simulink model "ppi_ctrl"  (R2020b)
settings: Solver=VariableStepAuto  StartTime=0.0  StopTime=10.0  RelTol=1e-3
values from neighbouring files (symbols this model uses):
  Ka = M_    [ppi_tuning.m]
  Kd = deltad1(2)*M_    [ppi_tuning.m]
  Ki = deltad1(3)*M_    [ppi_tuning.m]
  Kp = deltad2(1)/deltad1(3)    [ppi_tuning.m]    (also in script_ppi.m = double(Kp))
  q0 = [0 0 0 0]'    [script_ppi.m]
  traj_switch = 0    [script_ppi.m]
settings Model: Creator=lucas  LastModifiedBy=lucas

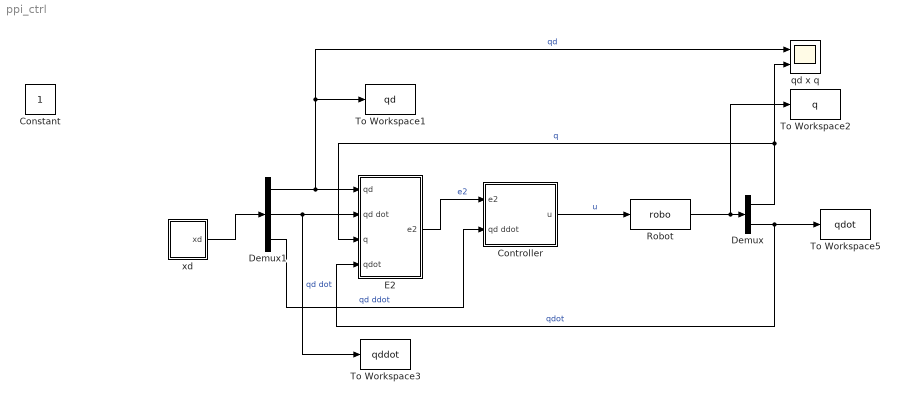
== system ppi_ctrl ==
  Controller : Subsystem
  Demux : Demux  Outputs=2
  Demux1 : Demux  Outputs=3
  E2 : Subsystem
  Robot : S-Function  FunctionName=robo  Parameters=q0  SFunctionDeploymentMode=off  EnableBusSupport=off  mask(Robot){xi=q0}
      mask prompts: xi "Condicao Inicial"
  To Workspace1 : ToWorkspace  VariableName=qd  SaveFormat=Timeseries  SampleTime=-1
  To Workspace2 : ToWorkspace  VariableName=q  SaveFormat=Timeseries  SampleTime=-1
  To Workspace3 : ToWorkspace  VariableName=qddot  SaveFormat=Timeseries  SampleTime=-1
  To Workspace5 : ToWorkspace  VariableName=qdot  SaveFormat=Timeseries  SampleTime=-1
  qd x q : Scope  NumInputPorts=2
  xd : Subsystem
  Constant : Constant  IOType=siggen
  wires:
  Demux/1 -> qd x q/2, E2/3(q)  "q"
  Demux1/1 -> To Workspace1/1, qd x q/1, E2/1(qd)  "qd"
  Demux1/2 -> To Workspace3/1, E2/2(qd dot)  "qd dot"
  Demux/2 -> To Workspace5/1, E2/4(qdot)  "qdot"
  E2/1(e2) -> Controller/1(e2)  "e2"
  Demux1/3 -> Controller/2(qd ddot)  "qd ddot"
  Controller/1(u) -> Robot/1  "u"
  Robot/1 -> To Workspace2/1, Demux/1
  xd/1(xd) -> Demux1/1

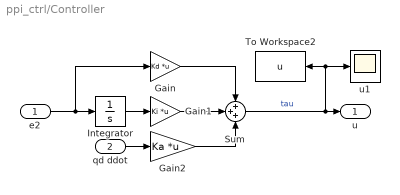
== system ppi_ctrl/Controller ==
  e2 : Inport
  qd ddot : Inport  Port=2
  Gain : Gain  Gain=Kd  Multiplication=Matrix(K*u)
  Gain1 : Gain  Gain=Ki  Multiplication=Matrix(K*u)
  Gain2 : Gain  Gain=Ka  Multiplication=Matrix(K*u)
  Integrator : Integrator
  Sum : Sum  Inputs=+++
  To Workspace2 : ToWorkspace  VariableName=u  SaveFormat=Timeseries  SampleTime=-1
  u1 : Scope
  u : Outport
  wires:
  Gain1/1 -> Sum/2
  qd ddot/1 -> Gain2/1
  Gain2/1 -> Sum/3
  Gain/1 -> Sum/1
  Integrator/1 -> Gain1/1
  e2/1 -> Gain/1, Integrator/1
  Sum/1 -> u1/1, To Workspace2/1, u/1  "tau"

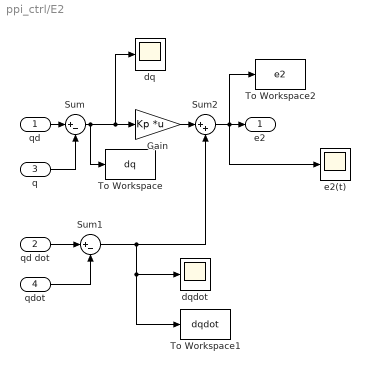
== system ppi_ctrl/E2 ==
  qd : Inport
  qd dot : Inport  Port=2
  q : Inport  Port=3
  qdot : Inport  Port=4
  Gain : Gain  Gain=Kp  Multiplication=Matrix(K*u)
  Sum : Sum  Inputs=|+-
  Sum1 : Sum  Inputs=|+-
  Sum2 : Sum  Inputs=|++
  To Workspace : ToWorkspace  VariableName=dq  SaveFormat=Timeseries  SampleTime=-1
  To Workspace1 : ToWorkspace  VariableName=dqdot  SaveFormat=Timeseries  SampleTime=-1
  To Workspace2 : ToWorkspace  VariableName=e2  SaveFormat=Timeseries  SampleTime=-1
  dq : Scope
  dqdot : Scope
  e2(t) : Scope
  e2 : Outport
  wires:
  Sum/1 -> To Workspace/1, dq/1, Gain/1
  Sum1/1 -> To Workspace1/1, dqdot/1, Sum2/2
  qdot/1 -> Sum1/2
  q/1 -> Sum/2
  Gain/1 -> Sum2/1
  qd/1 -> Sum/1
  qd dot/1 -> Sum1/1
  Sum2/1 -> e2(t)/1, To Workspace2/1, e2/1

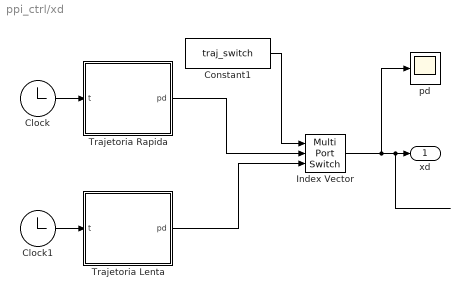
== system ppi_ctrl/xd ==
  Clock : Clock
  Clock1 : Clock
  Constant1 : Constant  Value=traj_switch
  Index Vector : MultiPortSwitch  DataPortOrder=Zero-based contiguous  Inputs=2  zeroidx=on
  Trajetoria Lenta : MATLAB Function  TreatAsAtomicUnit=on
  Trajetoria Rapida : MATLAB Function  TreatAsAtomicUnit=on
  pd : Scope
  xd : Outport
  wires:
  Trajetoria Lenta/1(pd) -> Index Vector/3
  Clock/1 -> Trajetoria Rapida/1(t)
  Constant1/1 -> Index Vector/1
  Trajetoria Rapida/1(pd) -> Index Vector/2
  Clock1/1 -> Trajetoria Lenta/1(t)
  Index Vector/1 -> pd/1, xd/1

== matlab function ppi_ctrl/xd/Trajetoria Lenta ==
  data: pd output; t input
function pd = fcn(t)
qd = [(-0.75*cos(pi*t/2))-0.75; (-0.75*cos(pi*t/2))+3.75];

qddot = [0.75*(pi/2)*sin(pi*t/2); 0.75*(pi/2)*sin(pi*t/2)];

qdddot = [0.75*(pi/2)^2*cos(pi*t/2); 0.75*(pi/2)^2*cos(pi*t/2)];

pd = [qd;qddot;qdddot];

== matlab function ppi_ctrl/xd/Trajetoria Rapida ==
  data: pd output; t input
function pd = fcn(t)
qd = [(-0.75*cos(pi*t))-0.75; (-0.75*cos(pi*t))+3.75];

qddot = [0.75*pi*sin(pi*t); 0.75*pi*sin(pi*t)];

qdddot = [0.75*pi^2*cos(pi*t); 0.75*pi^2*cos(pi*t)];

pd = [qd;qddot;qdddot];
